simulink model "model_task"  (R2025b)
settings: Solver=FixedStepDiscrete  StartTime=0.0  StopTime=15.0  FixedStep=0.1  RelTol=1e-3
settings Model: SimulationMode=rapid-accelerator  ExplicitPartitioning=on  Creator=jgillis  LastModifiedBy=jgillis
settings RTWCC: GenCodeOnly=on
settings GRTTargetCC: MatFileLogging=off

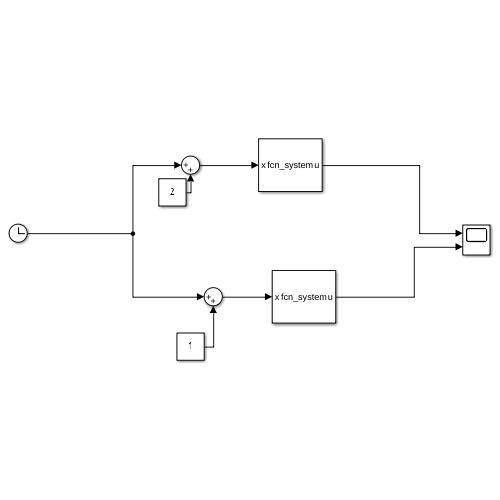
[thumbnail: Simulink's stored preview of the top-level diagram]
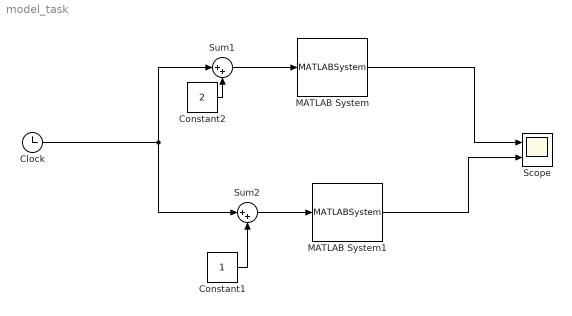
== system model_task ==
  Clock : Clock
  Constant1 : Constant
  Constant2 : Constant  Value=2
  MATLAB System : MATLABSystem  System=fcn_system  SimulateUsing=Code generation
      mask Type: fcn_system
  MATLAB System1 : MATLABSystem  System=fcn_system  SimulateUsing=Code generation
      mask Type: fcn_system
  Scope : Scope  NumInputPorts=2
      settings: ActiveDisplayYMinimum=-0.12500001250243464  ActiveDisplayYMaximum=11.125000112420905
  Sum1 : Sum  Inputs=|++
  Sum2 : Sum  Inputs=|++
  wires:
  Clock/1 -> Sum1/1, Sum2/1
  Constant1/1 -> Sum2/2
  Constant2/1 -> Sum1/2
  Sum1/1 -> MATLAB System/1
  MATLAB System/1 -> Scope/1
  Sum2/1 -> MATLAB System1/1
  MATLAB System1/1 -> Scope/2
